simulink model "igrf_wmm"  (Simulink 7.4)
settings: Solver=ode4  StartTime=0.0  StopTime=25000  FixedStep=.1  RelTol=1e-3
values from neighbouring files (symbols this model uses):
  Bstar = SGP4dragp    (= -3.5889e-05)    [constants_v16_integral_light_sun_sgp_igrf_power_13Dec2011.m]    (also in getOrbitData.m = SGP4dragp; sgp.m = modTLE(4))
  ddn0 = 6*2*pi*SGPdragp2/(1440^3)    (= 0)    [constants_v16_integral_light_sun_sgp_igrf_power_13Dec2011.m]    (also in getOrbitData.m = 6*2*pi*SGPdragp2/(1440^3); sgp.m = modTLE(3))
  dn0 = 2*2*pi*SGPdragp1/(1440^2)    (= -4.7632944169e-11)    [constants_v16_integral_light_sun_sgp_igrf_power_13Dec2011.m]    (also in getOrbitData.m = 2*2*pi*SGPdragp1/(1440^2); sgp.m = modTLE(2))
  equinox = datenum('21-Mar-2010 12:0:0')    [constants_v13.m]    (also in constants_v15.m; constants_v15_Pow.m = datenum('20-Mar-2015 12:0:0'); constants_v15_Pow_ss_error.m; constants_v16_integral_kartavya.m)
  err_SGP = 0    [constants_v16_integral_kartavya.m]    (also in constants_v16_integral_light_sun_sgp_igrf_power_13Dec2011.m)
  i0 = pi*orbInc/180    (= 1.72229090587)    [constants_v16_integral_light_sun_sgp_igrf_power_13Dec2011.m]    (also in getOrbitData.m = pi*orbInc/180; sgp.m = modTLE(5))
  M0 = pi*meanAno/180    (= 0)    [constants_v16_integral_light_sun_sgp_igrf_power_13Dec2011.m]    (also in getOrbitData.m = pi*meanAno/180; sgp.m = modTLE(9))
  n0 = 2*pi*meanMo/1440    [constants_v16_integral_light_sun_sgp_igrf_power_13Dec2011.m]    (also in getOrbitData.m; sgp.m = modTLE(10))
  Ohm0 = pi*rghtAsc/180    (= 3.21433797681)    [constants_v16_integral_light_sun_sgp_igrf_power_13Dec2011.m]    (also in getOrbitData.m = pi*rghtAsc/180; sgp.m = modTLE(6))
  revNo = 1    [constants_v16_integral_kartavya.m]    (also in constants_v16_integral_light_sun_sgp_igrf_power_13Dec2011.m; precalcs.m; sgp.m = modTLE(11))
  s_YEAR = sime(1) + (sime(2)*30 - 30 + sime(3))/365    [constants_v16_integral_kartavya.m]    (also in constants_v16_integral_light_sun_sgp_igrf_power_13Dec2011.m; precalcs.m = decyear(sime); virtuallabexpt3mag.m = decyear(sime))
  stperut = 1.00273790935    [constants_v16_integral_kartavya.m]    (also in constants_v16_integral_light_sun_sgp_igrf_power_13Dec2011.m; precalcs.m; virtuallabexpt3mag.m)
  t0 = (EpYear*meanYearDays + EpJD + EpTime)*1440    [constants_v16_integral_light_sun_sgp_igrf_power_13Dec2011.m]    (also in getOrbitData.m; sgp.m = modTLE(1))
  TLE_epoch = datenum('18-Oct-2015 10:30:0')    [constants_v15.m]    (also in constants_v16_integral_kartavya.m = datenum('18-Oct-2010 10:30:0'); constants_v16_integral_light_sun_sgp_igrf_power_13Dec2011.m = datenum('18-Oct-2010 10:30:0'); precalcs.m)
  today = datenum('18-Oct-2010 10:30:0')    [constants_v13.m]    (also in constants_v15.m; constants_v15_Pow.m = datenum('18-Oct-2015 10:30:0'); constants_v15_Pow_ss_error.m; constants_v16_integral_kartavya.m)
  w0 = pi*argPer/180    (= 0)    [constants_v16_integral_light_sun_sgp_igrf_power_13Dec2011.m]    (also in getOrbitData.m = pi*argPer/180; sgp.m = modTLE(8))
  W_EARTH_ROT = 2*pi/86400    (= 7.27220521664e-05)    [constants_v16_integral_kartavya.m]    (also in constants_v16_integral_light_sun_sgp_igrf_power_13Dec2011.m; precalcs.m; virtuallabexpt3mag.m)
undefined symbols (not defined in the file or in its folder): aeroassertmsg, agh, agh41, dgh, dgh41, Earth, WGS84
libraries: simulink x6, aerolibgravitysys x4, aerolibutil x2, aerolibtransform2 x2, aerolibconvert2 x2, dspmtrx3 x1
settings Model: Creator=satellite  LastModifiedBy=Jaideep

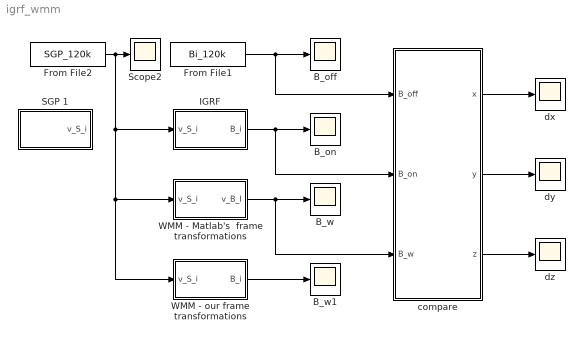
== system igrf_wmm ==
  B_off : Scope
      settings: YMin=-30000  YMax=35000  Decimation=6
  B_on : Scope
      settings: YMin=-35000  YMax=20000  Decimation=6
  B_w : Scope
      settings: YMin=-35000  YMax=20000  SaveName=ScopeData3  Decimation=6
  B_w1 : Scope
      settings: YMin=-35000  YMax=20000  SaveName=ScopeData7  Decimation=6
  From File1 : FromFile  FileName=Bi_120k
  From File2 : FromFile  FileName=SGP_120k
  "IGRF " : Subsystem
  SGP 1 : Subsystem
  Scope2 : Scope
      settings: YMin=-7e+006  YMax=8e+006  SaveName=ScopeData2  Decimation=6
  WMM - Matlab's  frame transformations : Subsystem
  WMM - our frame transformations : Subsystem
  compare : Stateflow chart
  dx : Scope
      settings: YMin=-30000  YMax=35000  SaveName=ScopeData4  Decimation=6
  dy : Scope
      settings: YMin=-35000  YMax=20000  SaveName=ScopeData5  Decimation=6
  dz : Scope
      settings: YMin=-35000  YMax=20000  SaveName=ScopeData6  Decimation=6
  wires:
  From File1/1 -> B_off/1, compare/1(B_off)
  From File2/1 -> Scope2/1, "IGRF "/1(v_S_i), WMM - Matlab's  frame transformations/1(v_S_i), WMM - our frame transformations/1(v_S_i)
  "IGRF "/1(B_i) -> B_on/1, compare/2(B_on)
  WMM - Matlab's  frame transformations/1(v_B_I) -> B_w/1, compare/3(B_w)
  compare/1(x) -> dx/1
  compare/2(y) -> dy/1
  compare/3(z) -> dz/1
  WMM - our frame transformations/1(B_i) -> B_w1/1

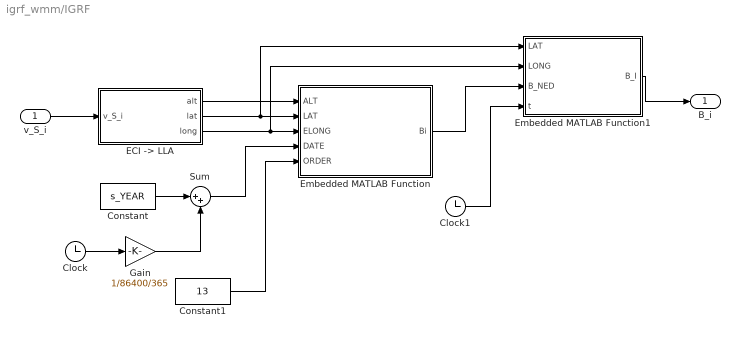
== system igrf_wmm/IGRF  ==
  v_S_i : Inport  OutDataType=fixdt(1, 16)  OutScaling=2^0
  Clock : Clock
      settings: Decimation=10
  Clock1 : Clock
      settings: Decimation=10
  Constant : Constant  Value=s_YEAR  OutDataType=fixdt(1, 16)  OutScaling=2^0
  Constant1 : Constant  Value=13  OutDataType=fixdt(1, 16)  OutScaling=2^0
  "ECI -> LLA" : Subsystem
  Embedded MATLAB Function : Stateflow chart
  Embedded MATLAB Function1 : Stateflow chart
  Gain : Gain  Gain=1/86400/365  ParameterDataType=fixdt(1, 16)  ParameterScaling=2^0  OutDataType=fixdt(1, 16)  OutScaling=2^0
  Sum : Sum  Inputs=|++  OutDataType=fixdt(1, 16)  OutScaling=2^0
  B_i : Outport  OutDataType=fixdt(1, 16)  OutScaling=2^0
  wires:
  v_S_i/1 -> "ECI -> LLA"/1(v_S_i)
  "ECI -> LLA"/1(alt) -> Embedded MATLAB Function/1(ALT)
  "ECI -> LLA"/2(lat) -> Embedded MATLAB Function/2(LAT), Embedded MATLAB Function1/1(LAT)
  "ECI -> LLA"/3(long) -> Embedded MATLAB Function/3(ELONG), Embedded MATLAB Function1/2(LONG)
  Clock/1 -> Gain/1
  Constant/1 -> Sum/1
  Gain/1 -> Sum/2
  Sum/1 -> Embedded MATLAB Function/4(DATE)
  Constant1/1 -> Embedded MATLAB Function/5(ORDER)
  Embedded MATLAB Function/1(Bi) -> Embedded MATLAB Function1/3(B_NED)
  Embedded MATLAB Function1/1(B_I) -> B_i/1
  Clock1/1 -> Embedded MATLAB Function1/4(t)

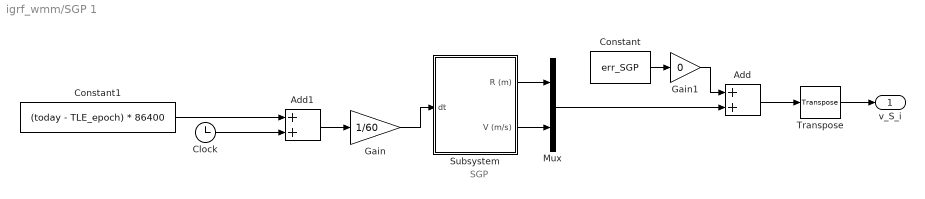
== system igrf_wmm/SGP 1 ==
  note: SGP
  Add : Sum  OutDataType=sfix(16)  OutScaling=2^-10
  Add1 : Sum  OutDataType=sfix(16)  OutScaling=2^-10
  Clock : Clock
      settings: Decimation=10
  Constant : Constant  Value=err_SGP  VectorParams1D=off  OutDataType=sfix(16)  OutScaling=2^0
  Constant1 : Constant  Value=(today - TLE_epoch) * 86400  VectorParams1D=off  OutDataType=sfix(16)  OutScaling=2^0
  Gain : Gain  Gain=1/60  ParameterDataType=sfix(16)  ParameterScaling=2^0  OutDataType=sfix(16)  OutScaling=2^0
  Gain1 : Gain  Gain=0  ParameterDataType=sfix(16)  ParameterScaling=2^0  OutDataType=sfix(16)  OutScaling=2^0
  Mux : Mux  Inputs=2
  Subsystem : Subsystem
  Transpose : dspmtrx3/Transpose  SystemSampleTime=-1  Hermitian=off  overflowFlag=off
  v_S_i : Outport  OutDataType=sfix(16)  OutScaling=2^0
  wires:
  Subsystem/1(R (m)) -> Mux/1
  Subsystem/2(V (m/s)) -> Mux/2
  Mux/1 -> Add/2
  Gain/1 -> Subsystem/1(dt)
  Constant/1 -> Gain1/1
  Add/1 -> Transpose/1
  Constant1/1 -> Add1/1
  Clock/1 -> Add1/2
  Add1/1 -> Gain/1
  Gain1/1 -> Add/1
  Transpose/1 -> v_S_i/1

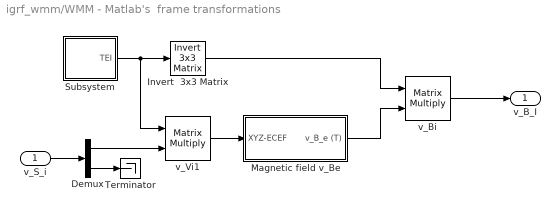
== system igrf_wmm/WMM - Matlab's  frame transformations ==
  v_S_i : Inport  OutDataType=sfix(16)  OutScaling=2^0
  Demux : Demux  Outputs=2
  Invert  3x3 Matrix : aerolibutil/Invert  3x3 Matrix  SystemSampleTime=-1
  Magnetic field v_Be : Subsystem
  Subsystem : Subsystem
  Terminator : Terminator
  v_Bi : Product  Multiplication=Matrix(*)  OutDataType=sfix(16)  OutScaling=2^0  RndMeth=Zero
  v_Vi1 : Product  Multiplication=Matrix(*)  OutDataType=sfix(16)  OutScaling=2^0  RndMeth=Zero
  v_B_I : Outport  OutDataType=sfix(16)  OutScaling=2^0
  wires:
  v_Bi/1 -> v_B_I/1
  Demux/1 -> v_Vi1/2
  v_S_i/1 -> Demux/1
  Demux/2 -> Terminator/1
  v_Vi1/1 -> Magnetic field v_Be/1(XYZ-ECEF)
  Subsystem/1(TEI) -> v_Vi1/1, Invert  3x3 Matrix/1
  Magnetic field v_Be/1("v_B_e (T) ") -> v_Bi/2
  Invert  3x3 Matrix/1 -> v_Bi/1

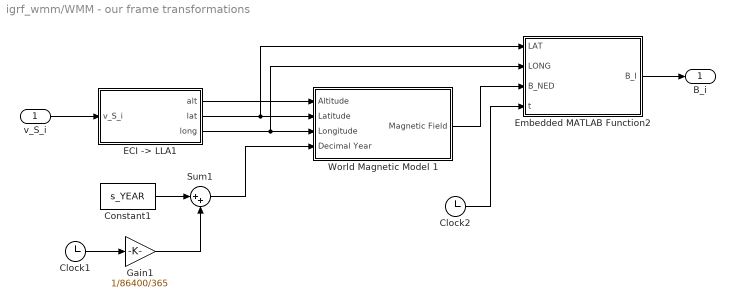
== system igrf_wmm/WMM - our frame transformations ==
  v_S_i : Inport  OutDataType=fixdt(1, 16)  OutScaling=2^0
  Clock1 : Clock
      settings: Decimation=10
  Clock2 : Clock
      settings: Decimation=10
  Constant1 : Constant  Value=s_YEAR  OutDataType=fixdt(1, 16)  OutScaling=2^0
  "ECI -> LLA1" : Subsystem
  Embedded MATLAB Function2 : Stateflow chart
  Gain1 : Gain  Gain=1/86400/365  ParameterDataType=fixdt(1, 16)  ParameterScaling=2^0  OutDataType=fixdt(1, 16)  OutScaling=2^0
  Sum1 : Sum  Inputs=|++  OutDataType=fixdt(1, 16)  OutScaling=2^0
  World Magnetic Model 1 : Subsystem  AncestorBlock=aerolibgravity2/World Magnetic Model 2005  mask(World Magnetic Model 2005){units=Metric (MKS), time_in=on, month=January, day=1, year=2005, action=Error, h_out=off, dec_out=off, inc_out=off, ti_out=off}
      mask prompts: time_in "Input decimal year"; action "Action for out of range input:"; h_out "Output horizontal intensity"; dec_out "Output declination"; inc_out "Output inclination"; ti_out "Output total intensity"
      mask help:
      | Calculate the Earth's magnetic field at a specific location and time using the World Magnetic Model (WMM). This model is valid for the year 2005 through the year 2010.
      |
      | The WMM-2005 can be found on the web at http://www.ngdc.noaa.gov/seg/WMM/DoDWMM.shtml and in "NOAA Technical Report: The US/UK World Magnetic Model for 2005-2010 ".
      |
      | Height is entered in length units of selected unit system. Latitude and longitude are entered in degrees.
      mask init:
      | [ports,dyear,maxdef,epoch,c,cd,fn,fm,snorm,k]=aeroicon('aeroblkwmm2005','icon');
      mask Help: eval('asbhelp');
      mask StyleString: popup(Metric (MKS)|English),checkbox,popup(January|February|March|April|May|June|July|August|September|October|November|December),popup(1|2|3|4|5|6|7|8|9|10|11|12|13|14|15|16|17|18|19|20|21|22|23|24|25|26|27|28|29|30|31),popup(2005|2006|2007|2008|2009|2010),popup(None|Warning|Error),checkbox,checkbox,checkbox,checkbox
      mask CallbackString: |aeroicon('aeroblkwmm');|aeroicon('aeroblkwmm');|aeroicon('aeroblkwmm');|aeroicon('aeroblkwmm');|||||
      mask Display:
      | port_label(ports(1).type,ports(1).port,ports(1).txt);
      | port_label(ports(2).type,ports(2).port,ports(2).txt,'texmode','on');
      | port_label(ports(3).type,ports(3).port,ports(3).txt,'texmode','on');
      | port_label(ports(4).type,ports(4).port,ports(4).txt);
      | port_label(ports(5).type,ports(5).port,ports(5).txt);
      | port_label(ports(6).type,ports(6).port,ports(6).txt);
      | port_label(ports(7).type,ports(7).port,ports(7).txt);
      | port_label(ports(8).type,ports(8).port,ports(8).txt);
      | port_label(ports(9).type,ports(9).port,ports(9).txt);
  B_i : Outport  OutDataType=fixdt(1, 16)  OutScaling=2^0
  wires:
  v_S_i/1 -> "ECI -> LLA1"/1(v_S_i)
  "ECI -> LLA1"/1(alt) -> World Magnetic Model 1/1(Altitude)
  "ECI -> LLA1"/2(lat) -> Embedded MATLAB Function2/1(LAT), World Magnetic Model 1/2(Latitude)
  "ECI -> LLA1"/3(long) -> Embedded MATLAB Function2/2(LONG), World Magnetic Model 1/3(Longitude)
  Clock1/1 -> Gain1/1
  Constant1/1 -> Sum1/1
  Gain1/1 -> Sum1/2
  Sum1/1 -> World Magnetic Model 1/4(Decimal Year)
  Embedded MATLAB Function2/1(B_I) -> B_i/1
  Clock2/1 -> Embedded MATLAB Function2/4(t)
  World Magnetic Model 1/1(Magnetic Field) -> Embedded MATLAB Function2/3(B_NED)

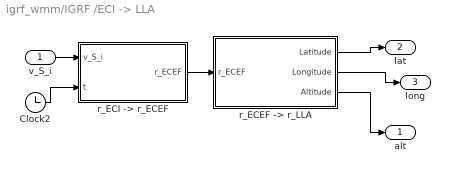
== system igrf_wmm/IGRF /ECI -> LLA ==
  v_S_i : Inport
  Clock2 : Clock
      settings: Decimation=10
  "r_ECEF -> r_LLA" : Stateflow chart
  "r_ECI -> r_ECEF" : Stateflow chart
  alt : Outport
  lat : Outport  Port=2
  long : Outport  Port=3
  wires:
  "r_ECEF -> r_LLA"/3(Altitude) -> alt/1
  "r_ECEF -> r_LLA"/2(Longitude) -> long/1
  v_S_i/1 -> "r_ECI -> r_ECEF"/1(v_S_i)
  "r_ECEF -> r_LLA"/1(Latitude) -> lat/1
  "r_ECI -> r_ECEF"/1(r_ECEF) -> "r_ECEF -> r_LLA"/1(r_ECEF)
  Clock2/1 -> "r_ECI -> r_ECEF"/2(t)

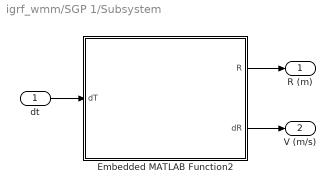
== system igrf_wmm/SGP 1/Subsystem ==
  dt : Inport
  Embedded MATLAB Function2 : Stateflow chart
  R (m) : Outport
  V (m/s) : Outport  Port=2
  wires:
  Embedded MATLAB Function2/1(R) -> R (m)/1
  dt/1 -> Embedded MATLAB Function2/1(dT)
  Embedded MATLAB Function2/2(dR) -> V (m/s)/1

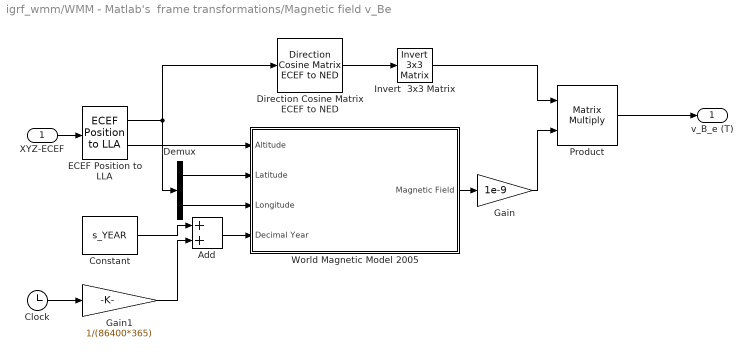
== system igrf_wmm/WMM - Matlab's  frame transformations/Magnetic field v_Be ==
  XYZ-ECEF : Inport  OutDataType=sfix(16)  OutScaling=2^0
  Add : Sum  OutDataType=sfix(16)  OutScaling=2^-10
  Clock : Clock
      settings: Decimation=10
  Constant : Constant  Value=s_YEAR  OutDataType=sfix(16)  OutScaling=2^0
  Demux : Demux  Outputs=2
  Direction Cosine Matrix ECEF to NED : aerolibtransform2/Direction Cosine Matrix ECEF to NED  SystemSampleTime=-1
  ECEF Position to LLA : aerolibtransform2/ECEF Position to LLA  SystemSampleTime=-1  units=Metric (MKS)  ptype=Earth (WGS84)  F=1/298.257223563  R=6378137
  Gain : Gain  Gain=1e-9  ParameterDataType=sfix(16)  ParameterScaling=2^0  OutDataType=sfix(16)  OutScaling=2^0
  Gain1 : Gain  Gain=1/(86400*365)  ParameterDataType=sfix(16)  ParameterScaling=2^0  OutDataType=sfix(16)  OutScaling=2^0
  Invert  3x3 Matrix : aerolibutil/Invert  3x3 Matrix  SystemSampleTime=-1
  Product : Product  Multiplication=Matrix(*)  OutDataType=sfix(16)  OutScaling=2^0  RndMeth=Zero
  World Magnetic Model 2005 : Subsystem  AncestorBlock=aerolibgravity2/World Magnetic Model 2005  mask(World Magnetic Model 2005){units=Metric (MKS), time_in=on, month=January, day=1, year=2005, action=Error, h_out=off, dec_out=off, inc_out=off, ti_out=off}
      mask prompts: time_in "Input decimal year"; action "Action for out of range input:"; h_out "Output horizontal intensity"; dec_out "Output declination"; inc_out "Output inclination"; ti_out "Output total intensity"
      mask help:
      | Calculate the Earth's magnetic field at a specific location and time using the World Magnetic Model (WMM). This model is valid for the year 2005 through the year 2010.
      |
      | The WMM-2005 can be found on the web at http://www.ngdc.noaa.gov/seg/WMM/DoDWMM.shtml and in "NOAA Technical Report: The US/UK World Magnetic Model for 2005-2010 ".
      |
      | Height is entered in length units of selected unit system. Latitude and longitude are entered in degrees.
      mask init:
      | [ports,dyear,maxdef,epoch,c,cd,fn,fm,snorm,k]=aeroicon('aeroblkwmm2005','icon');
      mask Help: eval('asbhelp');
      mask StyleString: popup(Metric (MKS)|English),checkbox,popup(January|February|March|April|May|June|July|August|September|October|November|December),popup(1|2|3|4|5|6|7|8|9|10|11|12|13|14|15|16|17|18|19|20|21|22|23|24|25|26|27|28|29|30|31),popup(2005|2006|2007|2008|2009|2010),popup(None|Warning|Error),checkbox,checkbox,checkbox,checkbox
      mask CallbackString: |aeroicon('aeroblkwmm');|aeroicon('aeroblkwmm');|aeroicon('aeroblkwmm');|aeroicon('aeroblkwmm');|||||
      mask Display:
      | port_label(ports(1).type,ports(1).port,ports(1).txt);
      | port_label(ports(2).type,ports(2).port,ports(2).txt,'texmode','on');
      | port_label(ports(3).type,ports(3).port,ports(3).txt,'texmode','on');
      | port_label(ports(4).type,ports(4).port,ports(4).txt);
      | port_label(ports(5).type,ports(5).port,ports(5).txt);
      | port_label(ports(6).type,ports(6).port,ports(6).txt);
      | port_label(ports(7).type,ports(7).port,ports(7).txt);
      | port_label(ports(8).type,ports(8).port,ports(8).txt);
      | port_label(ports(9).type,ports(9).port,ports(9).txt);
  "v_B_e (T) " : Outport  OutDataType=sfix(16)  OutScaling=2^0
  wires:
  Gain1/1 -> Add/2
  Clock/1 -> Gain1/1
  Add/1 -> World Magnetic Model 2005/4(Decimal Year)
  Constant/1 -> Add/1
  XYZ-ECEF/1 -> ECEF Position to LLA/1
  ECEF Position to LLA/1 -> Demux/1, Direction Cosine Matrix ECEF to NED/1
  ECEF Position to LLA/2 -> World Magnetic Model 2005/1(Altitude)
  Demux/1 -> World Magnetic Model 2005/2(Latitude)
  Demux/2 -> World Magnetic Model 2005/3(Longitude)
  Direction Cosine Matrix ECEF to NED/1 -> Invert  3x3 Matrix/1
  Invert  3x3 Matrix/1 -> Product/1
  Product/1 -> "v_B_e (T) "/1
  World Magnetic Model 2005/1(Magnetic Field) -> Gain/1
  Gain/1 -> Product/2

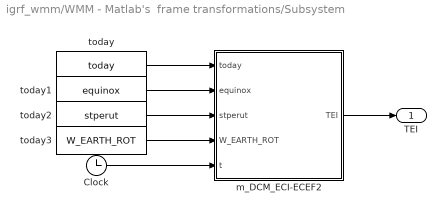
== system igrf_wmm/WMM - Matlab's  frame transformations/Subsystem ==
  Clock : Clock
      settings: Decimation=10
  m_DCM_ECI-ECEF2 : Stateflow chart
  today : Constant  Value=today  OutDataType=sfix(16)  OutScaling=2^0
  today1 : Constant  Value=equinox  OutDataType=sfix(16)  OutScaling=2^0
  today2 : Constant  Value=stperut  OutDataType=sfix(16)  OutScaling=2^0
  today3 : Constant  Value=W_EARTH_ROT  OutDataType=sfix(16)  OutScaling=2^0
  TEI : Outport
  wires:
  m_DCM_ECI-ECEF2/1(TEI) -> TEI/1
  Clock/1 -> m_DCM_ECI-ECEF2/5(t)
  today3/1 -> m_DCM_ECI-ECEF2/4(W_EARTH_ROT)
  today2/1 -> m_DCM_ECI-ECEF2/3(stperut)
  today1/1 -> m_DCM_ECI-ECEF2/2(equinox)
  today/1 -> m_DCM_ECI-ECEF2/1(today)

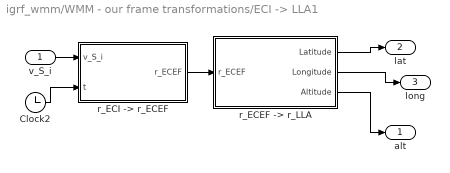
== system igrf_wmm/WMM - our frame transformations/ECI -> LLA1 ==
  v_S_i : Inport
  Clock2 : Clock
      settings: Decimation=10
  "r_ECEF -> r_LLA" : Stateflow chart
  "r_ECI -> r_ECEF" : Stateflow chart
  alt : Outport
  lat : Outport  Port=2
  long : Outport  Port=3
  wires:
  "r_ECEF -> r_LLA"/3(Altitude) -> alt/1
  "r_ECEF -> r_LLA"/2(Longitude) -> long/1
  v_S_i/1 -> "r_ECI -> r_ECEF"/1(v_S_i)
  "r_ECEF -> r_LLA"/1(Latitude) -> lat/1
  "r_ECI -> r_ECEF"/1(r_ECEF) -> "r_ECEF -> r_LLA"/1(r_ECEF)
  Clock2/1 -> "r_ECI -> r_ECEF"/2(t)

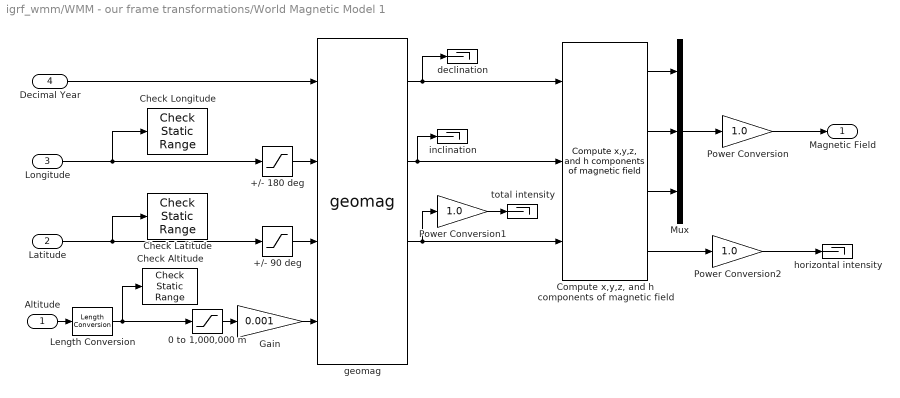
== system igrf_wmm/WMM - our frame transformations/World Magnetic Model 1 ==
  Altitude : Inport  OutDataType=sfix(16)  OutScaling=2^0
  Latitude : Inport  Port=2  OutDataType=sfix(16)  OutScaling=2^0
  Longitude : Inport  Port=3  OutDataType=sfix(16)  OutScaling=2^0
  Decimal Year : Inport  Port=4  OutDataType=sfix(16)  OutScaling=2^0
  +/- 180 deg : Saturate  UpperLimit=180.0  LowerLimit=-180.0  OutDataType=sfix(16)  OutScaling=2^0
  +/- 90 deg : Saturate  UpperLimit=90.0  LowerLimit=-90.0  OutDataType=sfix(16)  OutScaling=2^0
  0 to 1,000,000 m : Saturate  UpperLimit=1000000.0  LowerLimit=0  OutDataType=sfix(16)  OutScaling=2^0
  Check Altitude : simulink/Model Verification/Check  Static Range  Description=0 <= u <= 1000000  SystemSampleTime=-1  max=1000000  max_included=on  min=0  min_included=on  enabled=on  callback=aeroassertmsg('aeroblkwmm','alt');  stopWhenAssertionFail=on  export=off  icon=graphic
  Check Latitude : simulink/Model Verification/Check  Static Range  Description=-90 <= u <= 90  SystemSampleTime=-1  max=90  max_included=on  min=-90  min_included=on  enabled=on  callback=aeroassertmsg('aeroblkwmm','lat');  stopWhenAssertionFail=on  export=off  icon=graphic
  Check Longitude : simulink/Model Verification/Check  Static Range  Description=-180 <= u <= 180  SystemSampleTime=-1  max=180  max_included=on  min=-180  min_included=on  enabled=on  callback=aeroassertmsg('aeroblkwmm','lon');  stopWhenAssertionFail=on  export=off  icon=graphic
  "Compute x,y,z, and h components of magnetic field" : aerolibgravitysys/Compute x,y,z, and h components of magnetic field  SystemSampleTime=-1
  Gain : Gain  Gain=0.001  ParameterDataType=sfix(16)  ParameterScaling=2^0  OutDataType=sfix(16)  OutScaling=2^0  SaturateOnIntegerOverflow=on  OutDataTypeStr=Inherit: Same as input  ParamDataTypeStr=Inherit: Same as input
  Length Conversion : aerolibconvert2/Length Conversion  SystemSampleTime=-1  IU=m  OU=m
  Mux : Mux  Inputs=3
  Power Conversion : Gain  Gain=1.0  ParameterDataType=sfix(16)  ParameterScaling=2^0  OutDataType=sfix(16)  OutScaling=2^0  SaturateOnIntegerOverflow=on  OutDataTypeStr=Inherit: Same as input  ParamDataTypeStr=Inherit: Same as input
  Power Conversion1 : Gain  Gain=1.0  ParameterDataType=sfix(16)  ParameterScaling=2^0  OutDataType=sfix(16)  OutScaling=2^0  SaturateOnIntegerOverflow=on  OutDataTypeStr=Inherit: Same as input  ParamDataTypeStr=Inherit: Same as input
  Power Conversion2 : Gain  Gain=1.0  ParameterDataType=sfix(16)  ParameterScaling=2^0  OutDataType=sfix(16)  OutScaling=2^0  SaturateOnIntegerOverflow=on  OutDataTypeStr=Inherit: Same as input  ParamDataTypeStr=Inherit: Same as input
  declination : Terminator
  geomag : aerolibgravitysys/geomag  SystemSampleTime=-1
  horizontal intensity : Terminator
  inclination : Terminator
  total intensity : Terminator
  Magnetic Field : Outport  OutDataType=sfix(16)  OutScaling=2^0
  wires:
  0 to 1,000,000 m/1 -> Gain/1
  +/- 180 deg/1 -> geomag/2
  +/- 90 deg/1 -> geomag/3
  Power Conversion2/1 -> horizontal intensity/1
  Power Conversion1/1 -> total intensity/1
  Power Conversion/1 -> Magnetic Field/1
  Mux/1 -> Power Conversion/1
  geomag/1 -> declination/1, "Compute x,y,z, and h components of magnetic field"/1
  Gain/1 -> geomag/4
  Longitude/1 -> Check Longitude/1, +/- 180 deg/1
  Latitude/1 -> Check Latitude/1, +/- 90 deg/1
  geomag/3 -> Power Conversion1/1, "Compute x,y,z, and h components of magnetic field"/3
  geomag/2 -> inclination/1, "Compute x,y,z, and h components of magnetic field"/2
  Decimal Year/1 -> geomag/1
  "Compute x,y,z, and h components of magnetic field"/4 -> Power Conversion2/1
  "Compute x,y,z, and h components of magnetic field"/3 -> Mux/3
  "Compute x,y,z, and h components of magnetic field"/2 -> Mux/2
  "Compute x,y,z, and h components of magnetic field"/1 -> Mux/1
  Length Conversion/1 -> Check Altitude/1, 0 to 1,000,000 m/1
  Altitude/1 -> Length Conversion/1

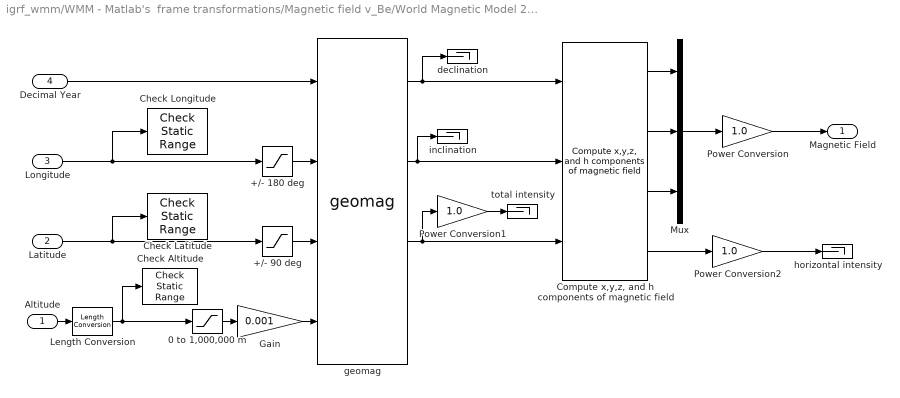
== system igrf_wmm/WMM - Matlab's  frame transformations/Magnetic field v_Be/World Magnetic Model 2005 ==
  Altitude : Inport  OutDataType=sfix(16)  OutScaling=2^0
  Latitude : Inport  Port=2  OutDataType=sfix(16)  OutScaling=2^0
  Longitude : Inport  Port=3  OutDataType=sfix(16)  OutScaling=2^0
  Decimal Year : Inport  Port=4  OutDataType=sfix(16)  OutScaling=2^0
  +/- 180 deg : Saturate  UpperLimit=180.0  LowerLimit=-180.0  OutDataType=sfix(16)  OutScaling=2^0
  +/- 90 deg : Saturate  UpperLimit=90.0  LowerLimit=-90.0  OutDataType=sfix(16)  OutScaling=2^0
  0 to 1,000,000 m : Saturate  UpperLimit=1000000.0  LowerLimit=0  OutDataType=sfix(16)  OutScaling=2^0
  Check Altitude : simulink/Model Verification/Check  Static Range  Description=0 <= u <= 1000000  SystemSampleTime=-1  max=1000000  max_included=on  min=0  min_included=on  enabled=on  callback=aeroassertmsg('aeroblkwmm','alt');  stopWhenAssertionFail=on  export=off  icon=graphic
  Check Latitude : simulink/Model Verification/Check  Static Range  Description=-90 <= u <= 90  SystemSampleTime=-1  max=90  max_included=on  min=-90  min_included=on  enabled=on  callback=aeroassertmsg('aeroblkwmm','lat');  stopWhenAssertionFail=on  export=off  icon=graphic
  Check Longitude : simulink/Model Verification/Check  Static Range  Description=-180 <= u <= 180  SystemSampleTime=-1  max=180  max_included=on  min=-180  min_included=on  enabled=on  callback=aeroassertmsg('aeroblkwmm','lon');  stopWhenAssertionFail=on  export=off  icon=graphic
  "Compute x,y,z, and h components of magnetic field" : aerolibgravitysys/Compute x,y,z, and h components of magnetic field  SystemSampleTime=-1
  Gain : Gain  Gain=0.001  ParameterDataType=sfix(16)  ParameterScaling=2^0  OutDataType=sfix(16)  OutScaling=2^0  SaturateOnIntegerOverflow=on  OutDataTypeStr=Inherit: Same as input  ParamDataTypeStr=Inherit: Same as input
  Length Conversion : aerolibconvert2/Length Conversion  SystemSampleTime=-1  IU=m  OU=m
  Mux : Mux  Inputs=3
  Power Conversion : Gain  Gain=1.0  ParameterDataType=sfix(16)  ParameterScaling=2^0  OutDataType=sfix(16)  OutScaling=2^0  SaturateOnIntegerOverflow=on  OutDataTypeStr=Inherit: Same as input  ParamDataTypeStr=Inherit: Same as input
  Power Conversion1 : Gain  Gain=1.0  ParameterDataType=sfix(16)  ParameterScaling=2^0  OutDataType=sfix(16)  OutScaling=2^0  SaturateOnIntegerOverflow=on  OutDataTypeStr=Inherit: Same as input  ParamDataTypeStr=Inherit: Same as input
  Power Conversion2 : Gain  Gain=1.0  ParameterDataType=sfix(16)  ParameterScaling=2^0  OutDataType=sfix(16)  OutScaling=2^0  SaturateOnIntegerOverflow=on  OutDataTypeStr=Inherit: Same as input  ParamDataTypeStr=Inherit: Same as input
  declination : Terminator
  geomag : aerolibgravitysys/geomag  SystemSampleTime=-1
  horizontal intensity : Terminator
  inclination : Terminator
  total intensity : Terminator
  Magnetic Field : Outport  OutDataType=sfix(16)  OutScaling=2^0
  wires:
  0 to 1,000,000 m/1 -> Gain/1
  +/- 180 deg/1 -> geomag/2
  +/- 90 deg/1 -> geomag/3
  Power Conversion2/1 -> horizontal intensity/1
  Power Conversion1/1 -> total intensity/1
  Power Conversion/1 -> Magnetic Field/1
  Mux/1 -> Power Conversion/1
  geomag/1 -> declination/1, "Compute x,y,z, and h components of magnetic field"/1
  Gain/1 -> geomag/4
  Longitude/1 -> Check Longitude/1, +/- 180 deg/1
  Latitude/1 -> Check Latitude/1, +/- 90 deg/1
  geomag/3 -> Power Conversion1/1, "Compute x,y,z, and h components of magnetic field"/3
  geomag/2 -> inclination/1, "Compute x,y,z, and h components of magnetic field"/2
  Decimal Year/1 -> geomag/1
  "Compute x,y,z, and h components of magnetic field"/4 -> Power Conversion2/1
  "Compute x,y,z, and h components of magnetic field"/3 -> Mux/3
  "Compute x,y,z, and h components of magnetic field"/2 -> Mux/2
  "Compute x,y,z, and h components of magnetic field"/1 -> Mux/1
  Length Conversion/1 -> Check Altitude/1, 0 to 1,000,000 m/1
  Altitude/1 -> Length Conversion/1

== matlab function IGRF /Embedded MATLAB Function ==
  data: ALT input double; Bi output double; LAT input double; ELONG input double; DATE input double; ORDER input double; agh parameter double; agh41 parameter double; dgh parameter double; dgh41 parameter double
function  Bi = igrf1(ALT,LAT,ELONG,DATE, ORDER, agh, agh41, dgh, dgh41)
%  MAGFD
%  Function to compute Earths magnetic field
%  and components: X,Y,Z,T for a given latitude
%  and longitude, date and altitude.
%  Uses MATLAB MAT files sh1900.mat to sh2010.mat in 5 yr
%  intervals. ONLY uses harmonic expansion to order 10 at present.
%
%  Usage: out=magfd(DATE,ITYPE,ALT,COLAT,ELONG);
%
%  DATE = date of survey (decimal years)
%  ITYPE=1 for geodetic coordinates (usual case)
%  ITYPE=2 for geocentric coordinates
%  ALT = (for ITYPE=1) altitude of survey relative to sealevel (km +ve up)
%  ALT = (for ITYPE=2) radial distance from center of earth in km
%  COLAT=90-latitude (decimal degrees)
%  ELONG=longitude of survey (decimal degrees)
%
%  Output array out contains components X,Y,Z,T in nanoteslas
%   X north component
%   Y east component     
%   Z vertical component +ve down
%   T total field magnitude
%
%  ref: IAGA, Division V, Working Group VMOD, 
%   The 10th generation International Geomagnetic 
%   Reference Field, Geophys. J. Int, 161, 561-565, 2005.
%
% Maurice A. Tivey March 1997
% Mod Dec 1999 (add igrf2000 and y2k compliance
% Mod Nov 2000 (use up to degree 10 sh coefficients)
% Mod Apr 2005 added 2005 coeffs
% Mod Sep 2006 some clean up and info added
% Mod Jan 2010 added 2010 coefficients
% http://deeptow.whoi.edu/matlab.html
% Copyright: Maurice A. Tivey, 2005
%  Woods Hole Oceanographic Institution

ITYPE = 1;
COLAT = 90- LAT;
CL = zeros(1,14);
SL = zeros(1,14);
P = zeros(1,104);
Q = zeros(1,104);
RR = 0;
FN = 0;

DGRF= 1000:5:2010;
igrfyear=2010;
% igrffile='sh2010';
% 
% pl=0;
% if DATE < 0, pl=1; end
% DATE=abs(DATE);
% Determine year for base DGRF to use.
% if DATE < igrfyear,
%     T =0;
%       BASE=fix(DATE-DGRF(1)); 
%       i=fix(BASE/5)+1;
%       BASE=DGRF(i);
% %       if pl==0,
% %           fprintf('Using DGRF base year %f \n',BASE);      
% %       end
%       eval(['load sh',num2str(BASE)])
%       % loads agh and agh41 but now need to get next epoch
%        iagh=agh;iagh41=agh41;
%       % figure out next epoch to load
%       if BASE < 1900, % a check to get pre-1900 estimates of gauss coeffs
%        eval(['load sh',num2str(BASE+25)])
%       else
%        eval(['load sh',num2str(DGRF(i+1))])
%       end
%        eagh=agh;eagh41=agh41;
%        dgh=(eagh-iagh)./5;dgh41=(eagh41-iagh41)./5;
%        agh=iagh;agh41=iagh41;
%        clear iagh iagh41 eagh eagh41
%        T = DATE - BASE;
% else
%       if pl==0,
%           fprintf('Using IGRF base year %f \n',igrfyear);       
%       end
%       eval(['load ',igrffile])   % load in igrf data file
      T     = DATE - igrfyear;
% end
% combine spherical harmonic coefficients from first 8 degrees 
% with degrees 9 thru 13 

 agh_full=[agh,agh41];
 dgh_full=[dgh,dgh41];
%
      D2R   = pi/180;
      R     = ALT;
      SLAT  = cos(COLAT*D2R);
      CLAT  = sin(COLAT*D2R);
      CL(1) = cos(ELONG*D2R);
      SL(1) = sin(ELONG*D2R);
      X     = 0.0;
      Y     = 0.0;
      Z     = 0.0;
      CD    = 1.0;
      SD    = 0.0;
      L     = 1;
      M     = 1;
      N     = 0;
      RE    = 6371.2; % Earth's mean radius
if ITYPE == 1  % CONVERSION FROM GEODETIC TO GEOCENTRIC COORDINATES
	%A2    = 40680925.;  % squared semi major axis
	%B2    = 40408588.;  % squared semi minor axis
    % WGS84
	A2    = 40680631.59; % 6378.137^2; % squared semi major axis
	B2    = 40408299.98; % 6356.7523142^2; % squared semi minor axis
	ONE   = A2*CLAT*CLAT;
	TWO   = B2*SLAT*SLAT;
	THREE = ONE + TWO;
	FOUR  = sqrt(THREE);
	R     = sqrt(ALT*(ALT + 2.0*FOUR) + (A2*ONE + B2*TWO)/THREE);
	CD    = (ALT + FOUR)/R;
	SD    = (A2 - B2)/FOUR*SLAT*CLAT/R;
	ONE   = SLAT;
	SLAT  = SLAT*CD - CLAT*SD;
	CLAT  = CLAT*CD +  ONE*SD;
end
% if geocentric coordinates desired then only need to define the following
	RATIO = RE/R;
%
%     COMPUTATION OF SCHMIDT QUASI-NORMAL COEFFICIENTS  P AND X(=Q)
%
      P(1)  = 2.0*SLAT;
      P(2)  = 2.0*CLAT;
      P(3)  = 4.5*SLAT*SLAT - 1.5;
      P(4)  = sqrt(27)*CLAT*SLAT;
      Q(1)  = -CLAT;
      Q(2)  =  SLAT;
      Q(3)  = -3.0*CLAT*SLAT;
      Q(4)  = sqrt(3)*(SLAT*SLAT - CLAT*CLAT);

NMAX=ORDER; % Max number of harmonic degrees
NPQ=(NMAX*(NMAX+3))/2;
for K=1:NPQ,
 if N < M 
	M     = 0;
	N     = N + 1;
	RR    = RATIO^(N + 2);
	FN    = N;
 end
 FM    = M;
 if K >= 5 %8,5,5
	if (M-N) == 0 %,7,6,7
		ONE   = sqrt(1.0 - 0.5/FM);
		J     = K - N - 1;
		P(K)  = (1.0 + 1.0/FM)*ONE*CLAT*P(J);
		Q(K)  = ONE*(CLAT*Q(J) + SLAT/FM*P(J));
		SL(M) = SL(M-1)*CL(1) + CL(M-1)*SL(1);
		CL(M) = CL(M-1)*CL(1) - SL(M-1)*SL(1);
	else
		ONE   = sqrt(FN*FN - FM*FM);
		TWO   = sqrt((FN - 1.0)^2 - FM*FM)/ONE;
		THREE = (2.0*FN - 1.0)/ONE;
		I     = K - N;
		J     = K - 2*N + 1;
		P(K)  = (FN + 1.0)*(THREE*SLAT/FN*P(I) - TWO/(FN - 1.0)*P(J));
		Q(K)  = THREE*(SLAT*Q(I) - CLAT/FN*P(I)) - TWO*Q(J);
	end
%
%     SYNTHESIS OF X, Y AND Z IN GEOCENTRIC COORDINATES
%
 end
 ONE   = (agh_full(L) + dgh_full(L)*T)*RR;

 if M == 0 %10,9,10
	X     = X + ONE*Q(K);
	Z     = Z - ONE*P(K);
	L     = L + 1;
 else
	TWO   = (agh_full(L+1) + dgh_full(L+1)*T)*RR;
	THREE = ONE*CL(M) + TWO*SL(M);
	X     = X + THREE*Q(K);
	Z     = Z - THREE*P(K);
	if CLAT > 0 %12,12,11
		Y = Y+(ONE*SL(M)-TWO*CL(M))*FM*P(K)/((FN + 1.0)*CLAT);
	else
		Y = Y + (ONE*SL(M) - TWO*CL(M))*Q(K)*SLAT;
	end
	L     = L + 2;
 end
	M     = M + 1;
end
%     CONVERSION TO COORDINATE SYSTEM SPECIFIED BY ITYPE

ONE   = X;
X     = X*CD +  Z*SD;
Z     = Z*CD - ONE*SD;
T     = sqrt(X*X + Y*Y + Z*Z);
Bi=[X,Y,Z];
%  END

== matlab function IGRF /ECI -> LLA/r_ECEF -> r_LLA ==
  data: r_ECEF input double; Latitude output double; Longitude output double; Altitude output double
function [Latitude, Longitude, Altitude] = fcn(r_ECEF)
%r_ECEF: ECEF position vector (in m)
%r_LLA: LLA postion vector (in rad, m)

% CHATI
% radius_earth = 6371000;
% r = norm(r_ECEF);
% x = r_ECEF(1);
% y = r_ECEF(2);
% z = r_ECEF(3);
% 
% lat = asin(z/r);
% long = atan2(y,x);
% if (long < 0)
%     long = long + 2*pi;
% end
% h = r - radius_earth;
% 
% Latitude = lat*180/pi; %deg
% Longitude = long*180/pi; %deg
% Altitude  = h/1000; %km
%r_LLA = [lat;long;h];

% 
% MATLAB
% L = ecef2lla(r_ECEF);
% Latitude = L(1); % deg
% Longitude = L(2); % deg
% Altitude = L(3)/1000; % km


% JAIDEEP
x = r_ECEF(1);
y = r_ECEF(2);
z = r_ECEF(3);

% wgs84model
f  = 1/298.257223563; % flattening
R =  6378137; % equatorial radius

% [phi, lambda, h] = ecef2geodetic(p(:,1), p(:,2), p(:,3), [R sqrt( 1 - ( 1 - f )^2 )]);
% Ellipsoid constants
% ellipsoid = [R sqrt( 1 - ( 1 - f )^2 )];
a  = R; % ellipsoid(1);       % Semimajor axis
e2 =  1 - ( 1 - f )^2; % ellipsoid(2) ^ 2;   % Square of first eccentricity
ep2 = e2 / (1 - e2);     % Square of second eccentricity
% f = 1 - sqrt(1 - e2);    % Flattening
b = a * (1 - f);         % Semiminor axis

% Longitude
lambda = atan2(y,x);

% Distance from Z-axis
rho = sqrt(x^2 + y^2);

% Bowring's formula for initial parametric (beta) and geodetic (phi) latitudes
beta = atan2(z, (1 - f) * rho);
phi = atan2(z   + b * ep2 * sin(beta).^3,...
            rho - a * e2  * cos(beta).^3);

% Fixed-point iteration with Bowring's formula
% (typically converges within two or three iterations)
betaNew = atan2((1 - f)*sin(phi), cos(phi));
count = 0;
while any(beta(:) ~= betaNew(:)) && count < 5
    beta = betaNew;
    phi = atan2(z   + b * ep2 * sin(beta).^3,...
                rho - a * e2  * cos(beta).^3);
    betaNew = atan2((1 - f)*sin(phi), cos(phi));
    count = count + 1;
end

% Calculate ellipsoidal height from the final value for latitude
sinphi = sin(phi);
N = a ./ sqrt(1 - e2 * sinphi.^2);
h = rho .* cos(phi) + (z + e2 * N .* sinphi) .* sinphi - N;

Latitude = phi*180/pi;
Longitude = lambda*180/pi;
Altitude = h/1000;  % km

== matlab function IGRF /Embedded MATLAB Function1 ==
  data: B_I output double; LAT input double; LONG input double; B_NED input double; today parameter double; equinox parameter double; t input double
function B_I = fcn(LAT, LONG, B_NED, today, equinox, t)
%#eml

stperut = 1.00273790935;    % siderial time = stperut * universal time
W_EARTH_ROT = 2*pi/86141;   % sidereal rotation angular velocity of earth, SI

ut_sec = (today - equinox)*24*60*60 + t; % universal time vector in sec
st_sec = stperut*ut_sec;    % sidereal time vector in sec

phi = st_sec*W_EARTH_ROT;            % sidereal time vector in rad

TEI = [ cos(phi) sin(phi) 0;
       -sin(phi) cos(phi) 0;
        0        0        1];


    
angles = [LAT LONG]*pi/180;

dcm = zeros(3,3,size(angles,1));  % dcmeceeftoned    
cang = cos( angles );
sang = sin( angles );

dcm(1,1,:) = -cang(:,2).*sang(:,1);
dcm(1,2,:) = -sang(:,2).*sang(:,1);
dcm(1,3,:) = cang(:,1);
dcm(2,1,:) = -sang(:,2);
dcm(2,2,:) = cang(:,2);
dcm(2,3,:) = 0.0;
dcm(3,1,:) = -cang(:,2).*cang(:,1);
dcm(3,2,:) = -sang(:,2).*cang(:,1);
dcm(3,3,:) = -sang(:,1);

B_ECEF = dcm'*B_NED';

B_I = TEI'*B_ECEF;

== matlab function IGRF /ECI -> LLA/r_ECI -> r_ECEF ==
  data: today parameter double; r_ECEF output double; equinox parameter double; v_S_i input double; t input double
function r_ECEF = fcn(today,equinox,v_S_i,t)
%u: position vector in ECI (in m)
%y: position vector in ECEF (in m)

r_I = v_S_i(1:3);

stperut = 1.00273790935;    % siderial time = stperut * universal time
W_EARTH_ROT = 2*pi/86141;   % sidereal rotation angular velocity of earth, SI

ut_sec = (today - equinox)*24*60*60 + t; % universal time vector in sec
st_sec = stperut*ut_sec;    % sidereal time vector in sec

phi = st_sec*W_EARTH_ROT;            % sidereal time vector in rad

TEI = [ cos(phi) sin(phi) 0;
       -sin(phi) cos(phi) 0;
        0        0        1];

r_ECEF = TEI*r_I;

== matlab function compare ==
  data: x output double; B_off input double; y output double; B_on input double; B_w input double; z output double
function [x,y,z] = f(B_off, B_on, B_w)
%#eml

x = [B_off.x; B_on.x; B_w.x];
y = [B_off.y; B_on.y; B_w.y];
z = [B_off.z; B_on.z; B_w.z];

== matlab function WMM - our frame transformations/ECI -> LLA1/r_ECEF -> r_LLA ==
  data: r_ECEF input double; Latitude output double; Longitude output double; Altitude output double
function [Latitude, Longitude, Altitude] = fcn(r_ECEF)
%r_ECEF: ECEF position vector (in m)
%r_LLA: LLA postion vector (in rad, m)

% CHATI
% radius_earth = 6371000;
% r = norm(r_ECEF);
% x = r_ECEF(1);
% y = r_ECEF(2);
% z = r_ECEF(3);
% 
% lat = asin(z/r);
% long = atan2(y,x);
% if (long < 0)
%     long = long + 2*pi;
% end
% h = r - radius_earth;
% 
% Latitude = lat*180/pi; %deg
% Longitude = long*180/pi; %deg
% Altitude  = h/1000; %km
%r_LLA = [lat;long;h];

% 
% MATLAB
% L = ecef2lla(r_ECEF);
% Latitude = L(1); % deg
% Longitude = L(2); % deg
% Altitude = L(3)/1000; % km


% JAIDEEP
x = r_ECEF(1);
y = r_ECEF(2);
z = r_ECEF(3);

% wgs84model
f  = 1/298.257223563; % flattening
R =  6378137; % equatorial radius

% [phi, lambda, h] = ecef2geodetic(p(:,1), p(:,2), p(:,3), [R sqrt( 1 - ( 1 - f )^2 )]);
% Ellipsoid constants
% ellipsoid = [R sqrt( 1 - ( 1 - f )^2 )];
a  = R; % ellipsoid(1);       % Semimajor axis
e2 =  1 - ( 1 - f )^2; % ellipsoid(2) ^ 2;   % Square of first eccentricity
ep2 = e2 / (1 - e2);     % Square of second eccentricity
% f = 1 - sqrt(1 - e2);    % Flattening
b = a * (1 - f);         % Semiminor axis

% Longitude
lambda = atan2(y,x);

% Distance from Z-axis
rho = sqrt(x^2 + y^2);

% Bowring's formula for initial parametric (beta) and geodetic (phi) latitudes
beta = atan2(z, (1 - f) * rho);
phi = atan2(z   + b * ep2 * sin(beta).^3,...
            rho - a * e2  * cos(beta).^3);

% Fixed-point iteration with Bowring's formula
% (typically converges within two or three iterations)
betaNew = atan2((1 - f)*sin(phi), cos(phi));
count = 0;
while any(beta(:) ~= betaNew(:)) && count < 5
    beta = betaNew;
    phi = atan2(z   + b * ep2 * sin(beta).^3,...
                rho - a * e2  * cos(beta).^3);
    betaNew = atan2((1 - f)*sin(phi), cos(phi));
    count = count + 1;
end

% Calculate ellipsoidal height from the final value for latitude
sinphi = sin(phi);
N = a ./ sqrt(1 - e2 * sinphi.^2);
h = rho .* cos(phi) + (z + e2 * N .* sinphi) .* sinphi - N;

Latitude = phi*180/pi;
Longitude = lambda*180/pi;
Altitude = h/1000;  % km

== matlab function WMM - our frame transformations/ECI -> LLA1/r_ECI -> r_ECEF ==
  data: today parameter double; r_ECEF output double; equinox parameter double; v_S_i input double; t input double
function r_ECEF = fcn(today,equinox,v_S_i,t)
%u: position vector in ECI (in m)
%y: position vector in ECEF (in m)

r_I = v_S_i(1:3);

stperut = 1.00273790935;    % siderial time = stperut * universal time
W_EARTH_ROT = 2*pi/86141;   % sidereal rotation angular velocity of earth, SI

ut_sec = (today - equinox)*24*60*60 + t; % universal time vector in sec
st_sec = stperut*ut_sec;    % sidereal time vector in sec

phi = st_sec*W_EARTH_ROT;            % sidereal time vector in rad

TEI = [ cos(phi) sin(phi) 0;
       -sin(phi) cos(phi) 0;
        0        0        1];

r_ECEF = TEI*r_I;

== matlab function WMM - our frame transformations/Embedded MATLAB Function2 ==
  data: B_I output double; LAT input double; LONG input double; B_NED input double; today parameter double; equinox parameter double; t input double
function B_I = fcn(LAT, LONG, B_NED, today, equinox, t)
%#eml

stperut = 1.00273790935;    % siderial time = stperut * universal time
W_EARTH_ROT = 2*pi/86141;   % sidereal rotation angular velocity of earth, SI

ut_sec = (today - equinox)*24*60*60 + t; % universal time vector in sec
st_sec = stperut*ut_sec;    % sidereal time vector in sec

phi = st_sec*W_EARTH_ROT;            % sidereal time vector in rad

TEI = [ cos(phi) sin(phi) 0;
       -sin(phi) cos(phi) 0;
        0        0        1];


    
angles = [LAT LONG]*pi/180;

dcm = zeros(3,3,size(angles,1));  % dcmeceeftoned    
cang = cos( angles );
sang = sin( angles );

dcm(1,1,:) = -cang(:,2).*sang(:,1);
dcm(1,2,:) = -sang(:,2).*sang(:,1);
dcm(1,3,:) = cang(:,1);
dcm(2,1,:) = -sang(:,2);
dcm(2,2,:) = cang(:,2);
dcm(2,3,:) = 0.0;
dcm(3,1,:) = -cang(:,2).*cang(:,1);
dcm(3,2,:) = -sang(:,2).*cang(:,1);
dcm(3,3,:) = -sang(:,1);

B_ECEF = dcm'*B_NED';

B_I = TEI'*B_ECEF;

== matlab function WMM - Matlab's frame transformations/Subsystem/m_DCM_ECI-ECEF2 ==
  data: TEI output double; today input double; equinox input double; stperut input double; W_EARTH_ROT input double; t input double
function TEI = fcn(today,equinox, stperut,W_EARTH_ROT,t)
% This block gives DCM for converting from ECI to ECEF frames
% inputs: today's date, equinox, sidereal time per unit time, angular velocity of earth's rotation, simulation time
% output: DCM

% 23hr 56m 4.09s per day

ut_sec = (today - equinox)*24*60*60 + t; % universal time in sec
st_sec = stperut*ut_sec;    % sidereal time in sec

phi = st_sec*W_EARTH_ROT;            % sidereal time in rad

TEI = [ cos(phi) sin(phi) 0;
       -sin(phi) cos(phi) 0;
        0        0        1];

== matlab function SGP 1/Subsystem/Embedded MATLAB Function2 ==
  data: t0 parameter double; dn0 parameter double; ddn0 parameter double; Bstar parameter double; i0 parameter double; Ohm0 parameter double; e0 parameter double; w0 parameter double; M0 parameter double; n0 parameter double; revNo parameter double; dT input double; R output double; dR output double
function [R, dR] = sgp(t0,dn0,ddn0,Bstar,i0,Ohm0,e0,w0,M0,n0,revNo,dT)
%This code is a matlab implementation of the SGP Fortran code in the
% Startrack report #3.
%
% The matlab code was derived mainly by porting and editing the
% FORTRAN routines in NORAD’s Spacetrack report #3.
% According to a statement in that report, the document is free
% of copyrights and open to unlimited public distribution.
%
% This matlab code is distributed under the same conditions
%
%
% Created 15/10-2001 by
% Klaus Krogsgaard & Torsten Lorentzen
% - - - - - - - - - - - - - - - - - - - - - - - - -
%
% SGP model for predicting orbit position.
%

% - - - - - - - - - - - - - - - - - - - - - - - - -
% Constants given by the modified NORAD TLE (all at epoch)
% - - - - - - - - - - - - - - - - - - - - - - - - -


% t0 = modTLE(1);
% dn0 = modTLE(2); % first time derivative of the mean motion
% ddn0 = modTLE(3); % second time derivative of mean motion
% Bstar = modTLE(4); % Drag parameter
% i0 = modTLE(5); % inclination
% Ohm0 = modTLE(6); % right ascension of the ascending node
% e0 = modTLE(7); % eccentricity
% w0 = modTLE(8); % argument of perigee
% M0 = modTLE(9); % mean anormaly
% n0 = modTLE(10); % mean motion
% revNo = modTLE(11); % Number of revolutions before epoch
% - - - - - - - - - - - - - - - - - - - - - - - - -
% Other constants
% - - - - - - - - - - - - - - - - - - - - - - - - -
GM = 398603 * 10^9;
er = 6378.135;
ke = 0.0743669161; %converted to er/min ^3/2
% aE = 6378160; % equatorial radius of the Earth
aE = 1;% give result in Earth radii
min_per_day = 1440;
sec_per_day = 86400;
km_per_er = er;
J2 = 5.413080*10^-4 * 2; % second gravitational zonal harmonic of the Earth
J3 = -0.253881*10^-5; % third gravitational zonal harmonic of the Earth
J4 = -0.62098875*10^-6 * 8/3; % fourth gravitational zonal harmonic of the Earth
% - - - - - - - - - - - - - - - - - - - - - - - - -
% Local constants
% - - - - - - - - - - - - - - - - - - - - - - - - -
a1 = (ke/n0)^(2/3);
delta1 = 3/4 * J2 * (aE/a1)^2 * (3*((cos(i0))^2)-1)/((1-e0^2)^(3/2));
a0 = a1 * (1 - 1/3*delta1 - delta1^2 - 134/81*delta1^3);
p0 = a0 * (1 - e0^2);
q0 = a0 * (1-e0);
L0 = M0 + w0 + Ohm0;
dOhm = - (3/2) * J2 * (aE/p0)^2 * n0 * cos(i0);
dw = (3/4) * J2 * (aE/p0)^2 * n0 * (5*(cos(i0))^2-1);
% - - - - - - - - - - - - - - - - - - - - - - - - -
% Secular effects of drag and gravitation
% - - - - - - - - - - - - - - - - - - - - - - - - -
a = a0 * ( n0 ./ (n0 + 2*(dn0/2)*(dT) + 3*(ddn0/6)*dT.^2)).^(2/3); % vector
e = zeros(1,length(dT)); % vector
for i=1:length(a)
if ( a(i)>q0 )
e(i) = 1 - q0/a(i);
else
e(i) = 10^-6;
end;
end;
p = a .* (1-e.^2); % vector
OhmS0 = Ohm0 + dOhm * dT; % vector
wS0 = w0 + dw * (dT); % vector
Ls = mod(L0 + (n0 + dw + dOhm)*(dT) + dn0/2 * (dT).^2 + ddn0/6 * (dT).^3,2*pi); % vector
% - - - - - - - - - - - - - - - - - - - - - - - - -
% Long period periodic effects
% - - - - - - - - - - - - - - - - - - - - - - - - -
axNSL = e .* cos(wS0); % vector
ayNSL = e .* sin(wS0) - 1/2 * J3/J2 * aE./p * sin(i0); % vector
L = mod(Ls - 1/4 * J3/J2 * aE./p .* axNSL * sin(i0) * (3+5*cos(i0))/(1+cos(i0)),2*pi); % vector
% - - - - - - - - - - - - - - - - - - - - - - - - -
% Iteration
% - - - - - - - - - - - - - - - - - - - - - - - - -
tol = 10^-8;
U = mod(L - OhmS0,2*pi); % vector
Ew1 = U; % vector
Ew2 = Ew1; % vector
dEw = (U - ayNSL.*cos(Ew1) + axNSL.*sin(Ew1) - Ew1) ./ (-ayNSL.*sin(Ew1) - axNSL.*cos(Ew1) + 1); % vector
for i=1:length(dEw)
if abs(dEw(i)) > 1
Ew2(i) = Ew1(i) + sign(dEw(i)); %vector
else
Ew2(i) = Ew1(i) + dEw(i);
end;
end;
for i=1:length(Ew1)
while abs(dEw(i))>tol
Ew1(i) = Ew2(i);
dEw(i) = (U(i) - ayNSL(i).*cos(Ew1(i)) + axNSL(i).*sin(Ew1(i)) - Ew1(i)) ./ ...
(-ayNSL(i).*sin(Ew1(i)) - axNSL(i).*cos(Ew1(i)) + 1);
if abs(dEw(i)) > 1
Ew2(i) = Ew1(i) + sign(dEw(i)); %vector
else
Ew2(i) = Ew1(i) + dEw(i);
end;
end;
end;
ecosE = axNSL.*cos(Ew2) + ayNSL.*sin(Ew2); % vector
esinE = axNSL.*sin(Ew2) - ayNSL.*cos(Ew2); % vector
SQeL = axNSL.^2 + ayNSL.^2; % vector
pL = a.*(1 - SQeL); % vector
r = a.*(1 - ecosE); % vector
dr = ke * sqrt(a)./r .* esinE; % vector
rdv = ke * sqrt(pL)./r; % vector
sinu = a./r .* (sin(Ew2) - ayNSL - axNSL.*esinE./(1+sqrt(1-SQeL))); % vector
cosu = a./r .* (cos(Ew2) - axNSL + ayNSL.*esinE./(1+sqrt(1-SQeL))); % vectro
u = mod(atan2( sinu,cosu ),2*pi); % vector
% - - - - - - - - - - - - - - - - - - - - - - - - -
% Short term perturbations
% - - - - - - - - - - - - - - - - - - - - - - - - -
rk = r + 1/4 * J2 * aE^2./pL * (sin(i0))^2 .* cos(2*u); % vector
uk = u - 1/8 * J2 * (aE./pL).^2 * (7 * (cos(i0))^2 - 1) .* sin(2*u); % vector
Ohmk = OhmS0 + 3/4 * J2 * (aE./pL).^2 * cos(i0) .* sin(2*u); % vector
ik = i0 + 3/4 * J2 * (aE./pL).^2 * sin(i0) * cos(i0) .* cos(2*u); % vector
% - - - - - - - - - - - - - - - - - - - - - - - - -
% Unit orientation vectors
% - - - - - - - - - - - - - - - - - - - - - - - - -
R = zeros(length(uk),3); % vector
dR = zeros(length(uk),3); % vector
for i=1:length(uk)
    M_vec = [ -sin(Ohmk(i))*cos(ik(i)) cos(Ohmk(i))*cos(ik(i)) sin(ik(i)) ]; % vector
N_vec = [ cos(Ohmk(i)) sin(Ohmk(i)) 0 ]; % vector
U_vec = M_vec * sin(uk(i)) + N_vec * cos(uk(i)); % vector
V_vec = M_vec * cos(uk(i)) - N_vec * sin(uk(i)); % vector
% - - - - - - - - - - - - - - - - - - - - - - - - -
% Position and velocity
% - - - - - - - - - - - - - - - - - - - - - - - - -
R(i,:) = rk(i) * U_vec; % vector
dR(i,:) = dr(i) * U_vec + rdv(i) * V_vec; % vector
end;
% - - - - - - - - - - - - - - - - - - - - - - - - -
% Transforming position to Cartesian coordinates in kilometers and velocity to kilometers/sec
% - - - - - - - - - - - - - - - - - - - - - - - - -
R = R * km_per_er /aE;
R = R * 1000; % km to m
dR = dR * km_per_er / aE * min_per_day / sec_per_day;
dR = dR * 1000; % km/s to m/s
